simulink model "mlf_median"  (R2015b)
settings: Solver=FixedStepDiscrete  SolverMode=SingleTasking  StartTime=0.0  StopTime=10  RelTol=1e-3
libraries: simulink x2, dspstat3 x1
settings Model: Creator=at-mt  LastModifiedBy=amatsumo
settings DataIOCC: SaveFormat=Array  SignalLoggingSaveFormat=ModelDataLogs  SaveOutput=off  SignalLogging=off  SaveTime=off
settings OptimizationCC: BlockReduction=off  ConditionallyExecuteInputs=off  DefaultParameterBehavior=Inlined  ExpressionDepthLimit=2147483647
settings DebuggingCC: AlgebraicLoopMsg=error  UnderspecifiedInitializationDetection=Classic  MergeDetectMultiDrivingBlocksExec=none  SolverPrmCheckMsg=warning  SingleTaskRateTransMsg=error  FcnCallInpInsideContextMsg=UseLocalSettings  StateNameClashWarn=warning
settings HardwareCC: ProdBitPerPointer=32  ProdLargestAtomicFloat=None  ProdIntDivRoundTo=Undefined  ProdEndianess=Unspecified  ProdWordSize=32  ProdHWDeviceType=ASIC/FPGA->ASIC/FPGA  ProdEqTarget=off
settings SFSimCC: SFSimEcho=off  SimParseCustomCode=off
settings GRTTargetCC: GeneratePreprocessorConditionals=Disable all  CombineOutputUpdateFcns=off  GRTInterface=on
settings ConfigComp: CovModelRefEnable=Off  CovSFcnEnable=off

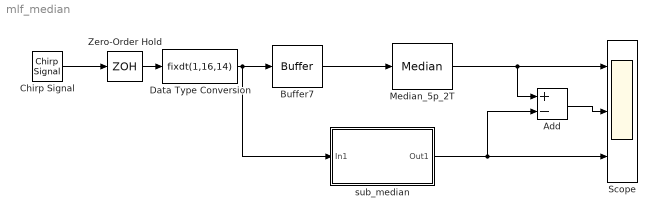
== system mlf_median ==
  Add : Sum  Inputs=+-
  Buffer7 : Buffer  N=5  V=4  TreatMby1Signals=One channel
  Chirp Signal : simulink/Sources/Chirp Signal  f1=10  T=10  f2=500
  Data Type Conversion : DataTypeConversion  OutDataTypeStr=fixdt(1,16,14)
  Median_5p_2T : dspstat3/Median  sortAlg=Quick sort  directionMode=Each column  dimension=1  outputDataTypeStr=Inherit: Same as accumulator  outputLastDataTypeStr=Inherit: Same as accumulator  outputMin=[]  outputMax=[]  accumDataTypeStr=Inherit: Same as product output  accumLastDataTypeStr=Inherit: Same as product output  roundingMode=Floor  overflowMode=off
      settings: allowOverrides=off
  Scope : Scope  NumInputPorts=3
  Zero-Order Hold : ZeroOrderHold  SampleTime=1/1000
  sub_median : Subsystem
  wires:
  Chirp Signal/1 -> Zero-Order Hold/1
  Zero-Order Hold/1 -> Data Type Conversion/1
  Median_5p_2T/1 -> Add/1, Scope/1
  Add/1 -> Scope/2
  Buffer7/1 -> Median_5p_2T/1
  sub_median/1(Out1) -> Add/2, Scope/3
  Data Type Conversion/1 -> Buffer7/1, sub_median/1(In1)

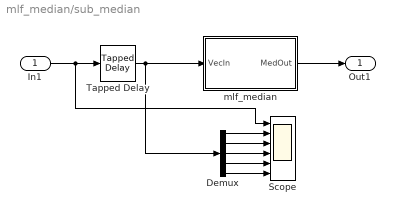
== system mlf_median/sub_median ==
  In1 : Inport
  Demux : Demux  Outputs=5
  Scope : Scope  NumInputPorts=6
  Tapped Delay : simulink/Discrete/Tapped Delay  vinit=0.0  samptime=-1  NumDelays=4  DelayOrder=Newest  includeCurrent=on
  mlf_median : MATLAB Function  TreatAsAtomicUnit=on
  Out1 : Outport
  wires:
  Tapped Delay/1 -> mlf_median/1(VecIn), Demux/1
  In1/1 -> Tapped Delay/1, Scope/1
  mlf_median/1(MedOut) -> Out1/1
  Demux/1 -> Scope/2
  Demux/2 -> Scope/3
  Demux/3 -> Scope/4
  Demux/4 -> Scope/5
  Demux/5 -> Scope/6

== matlab function mlf_median/sub_median/mlf_median ==
  settings: fimath=|
      | fimath(...
      | 'RoundMode', 'floor',...
      | 'OverflowMode', 'wrap',...
      | 'ProductMode', 'KeepLSB', 'ProductWordLength', 16,...
      | 'SumMode', 'KeepLSB', 'SumWordLength', 16,...
      | 'CastBeforeSum', true)
  data: VecIn input; MedOut output
function MedOut = fcn(VecIn)
% median filter
InputLength = 5;
for n = uint8(1:length(VecIn))
    for m = uint8(1:length(VecIn) - 1)
        if VecIn(m) > VecIn(m+1)
            tmp = VecIn(m+1);
            VecIn(m+1) = VecIn(m);
            VecIn(m) = tmp;
        end
    end
end

MedOut = VecIn(round(InputLength/2));
